simulink model "simulinkquestao_2"  (R2020a)
settings: Solver=FixedStepAuto  StartTime=0.0  StopTime=7  FixedStep=1e-4  RelTol=1e-3
undefined symbols (not defined in the file): A, B, C, K_realimentacao, L_observador
settings Model: OrderedModelArguments=off  Creator=Dylan  LastModifiedBy=Dylan Soares

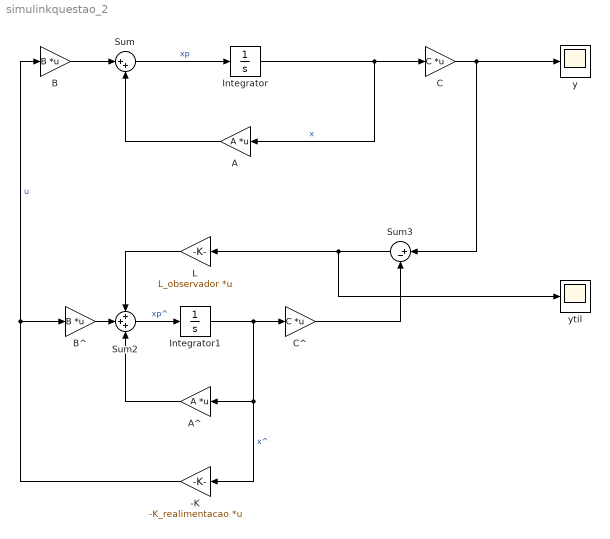
== system simulinkquestao_2 ==
  -K : Gain  Gain=-K_realimentacao  Multiplication=Matrix(K*u) (u vector)
  A : Gain  Gain=A  Multiplication=Matrix(K*u) (u vector)
  A^ : Gain  Gain=A  Multiplication=Matrix(K*u) (u vector)
  B : Gain  Gain=B  Multiplication=Matrix(K*u)
  B^ : Gain  Gain=B  Multiplication=Matrix(K*u)
  C : Gain  Gain=C  Multiplication=Matrix(K*u) (u vector)
  C^ : Gain  Gain=C  Multiplication=Matrix(K*u) (u vector)
  Integrator : Integrator  InitialCondition=[1,0,0,0]
  Integrator1 : Integrator  InitialCondition=[-1,0,0,0]
  L : Gain  Gain=L_observador  Multiplication=Matrix(K*u) (u vector)
  Sum : Sum  Inputs=|++
  Sum2 : Sum  Inputs=+++
  Sum3 : Sum  Inputs=|+-
  y : Scope
  ytil : Scope
  wires:
  A/1 -> Sum/2
  Integrator/1 -> C/1, A/1  "x"
  B/1 -> Sum/1
  Sum/1 -> Integrator/1  "xp"
  -K/1 -> B/1, B^/1  "u"
  Integrator1/1 -> -K/1, A^/1, C^/1  "x^"
  C^/1 -> Sum3/2
  Sum2/1 -> Integrator1/1  "xp^"
  C/1 -> y/1, Sum3/1
  A^/1 -> Sum2/3
  B^/1 -> Sum2/2
  L/1 -> Sum2/1
  Sum3/1 -> ytil/1, L/1
